simulink model "scouts"  (R2018a)
settings: Solver=VariableStepAuto  StartTime=0.0  StopTime=500  FixedStep=0.01  MaxStep=0.01  RelTol=1e-5
undefined symbols (not defined in the file or in its folder): sigbuilder_block
libraries: simulink x2
settings Model: Creator=daniel  LastModifiedBy=blond
settings SolverCC: ZeroCrossAlgorithm=Adaptive  AlgebraicLoopSolver=LineSearch
settings DebuggingCC: MaxConsecutiveZCsMsg=warning

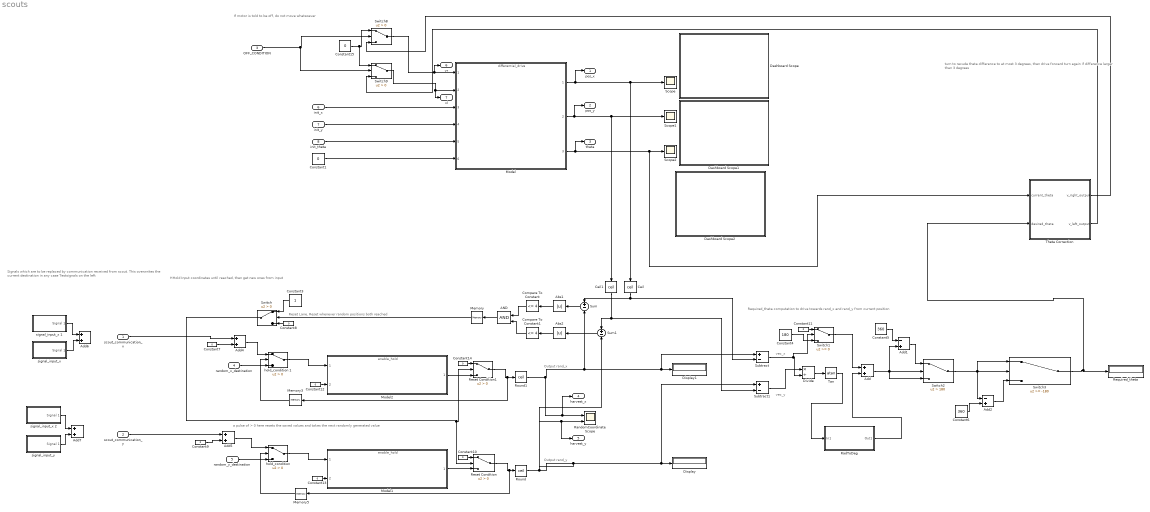
== system scouts ==
  note: If motor is told to be off, do not move whatsoever
  note: Signals which are to be replaced
      | by communication received
      | from scout. This overwrites the
      | current destination in any case
      |
      | Testsignals on the left
  note: turn to recude theta difference to at
      | most 3 degrees, then drive forward
      | turn again if difference larger than
      | 3 degrees
  note: Required_theta computation to drive towards rand_x and rand_y from current position
  note: vec_y
  note: Reset Lane, Reset whenever random positions both reached
  note: a pulse of > 0 here resets the saved values and takes the next randomly generated value
  note: Output rand_x
  note: HHold Input coordinates until reached, then get new ones from input
  note: Output rand_y
  note: vec_x
  "scout_communication_x " : Inport
  scout_communication_y : Inport  Port=2
  "OFF_CONDITION " : Inport  Port=3
  random_x_destination : Inport  Port=4
  random_y_destination : Inport  Port=5
  "init_x " : Inport  Port=6
  init_y : Inport  Port=7
  "init_theta " : Inport  Port=8
  AND : Logic  IconShape=distinctive  AllPortsSameDT=off  OutDataTypeStr=boolean
  Abs1 : Abs
  Abs2 : Abs
  Add{,4..7} (5 alike) : Sum
  Add1 : Sum  Inputs=-+
  Add2 : Sum  Inputs=-+
  Ceil : Rounding  Operator=ceil
  Ceil1 : Rounding  Operator=ceil
  Compare To Constant : simulink/Logic and Bit Operations/Compare To Constant  relop=<=  const=4  OutDataTypeStr=boolean
  Compare To Constant1 : simulink/Logic and Bit Operations/Compare To Constant  relop=<=  const=4  OutDataTypeStr=boolean
  Constant{1,7..15} (10 alike) : Constant  Value=0
  Constant3 : Constant
  Constant4 : Constant  Value=180
  Constant5 : Constant  Value=360
  Constant6 : Constant  Value=360
  Dashboard Scope : Subsystem  DialogController=hmiCreateDDGDialog  IsWebBlock=on  mask(MWDashboardBlock){webBlockId=28513450-4590-42fc-ab75-f58e69578865, webBlockType=sdiscope, ShowInitialText=on, HMISrcModelName=scouts}
      mask prompts: webBlockId "WebBlock Id"; webBlockType "WebBlock Type"; HMISrcModelName "Source Model"
      mask help: SimulinkHMI:dialogs:HMIScopeDialogDesc
      mask Help: helpview([docroot '/mapfiles/simulink.map'], 'hmi_scope')
      mask Display:
      | if strcmp(get_param(bdroot(gcb),'BlockDiagramType'), 'library')
      |     image([(matlabroot) '/toolbox/simulink/hmi/icons/DashboardScope.png']);
      | end
  Dashboard Scope1 : Subsystem  DialogController=hmiCreateDDGDialog  IsWebBlock=on  mask(MWDashboardBlock){webBlockId=3c51b7a5-38a5-4713-bbf7-871b8fd5eea3, webBlockType=sdiscope, ShowInitialText=on, HMISrcModelName=scouts}
      mask prompts: webBlockId "WebBlock Id"; webBlockType "WebBlock Type"; HMISrcModelName "Source Model"
      mask help: SimulinkHMI:dialogs:HMIScopeDialogDesc
      mask Help: helpview([docroot '/mapfiles/simulink.map'], 'hmi_scope')
      mask Display:
      | if strcmp(get_param(bdroot(gcb),'BlockDiagramType'), 'library')
      |     image([(matlabroot) '/toolbox/simulink/hmi/icons/DashboardScope.png']);
      | end
  Dashboard Scope2 : Subsystem  DialogController=hmiCreateDDGDialog  IsWebBlock=on  mask(MWDashboardBlock){webBlockId=0047718c-4f1b-48ee-af11-e80bd18439e0, webBlockType=sdiscope, ShowInitialText=on, HMISrcModelName=scouts}
      mask prompts: webBlockId "WebBlock Id"; webBlockType "WebBlock Type"; HMISrcModelName "Source Model"
      mask help: SimulinkHMI:dialogs:HMIScopeDialogDesc
      mask Help: helpview([docroot '/mapfiles/simulink.map'], 'hmi_scope')
      mask Display:
      | if strcmp(get_param(bdroot(gcb),'BlockDiagramType'), 'library')
      |     image([(matlabroot) '/toolbox/simulink/hmi/icons/DashboardScope.png']);
      | end
  Display : Display
  Display1 : Display
  Divide : Product  Inputs=*/
  Memory : Memory
  Memory3 : Memory  InheritSampleTime=on
  Memory5 : Memory  InheritSampleTime=on
  Model : ModelReference  ModelNameDialog=differential_drive.slx  SimulationMode=Normal  ModelReferenceVersion=1.286
  Model1 : ModelReference  ModelNameDialog=enable_hold.slx  SimulationMode=Normal  ModelReferenceVersion=1.281
  Model2 : ModelReference  ModelNameDialog=enable_hold.slx  SimulationMode=Normal  ModelReferenceVersion=1.281
  RadToDeg : Subsystem
  "RandomCoordinate Scope " : Scope  NumInputPorts=2
  Required_theta : Display
  Reset Condition : Switch  Criteria=u2 > Threshold
  Reset Condition1 : Switch  Criteria=u2 > Threshold
  Round : Rounding  Operator=ceil
  Round1 : Rounding  Operator=ceil
  Scope : Scope
  Scope1 : Scope
  Scope2 : Scope
  Subtract : Sum  Inputs=+-
  Subtract1 : Sum  Inputs=+-
  Sum : Sum  Inputs=+-
  Sum1 : Sum  Inputs=+-
  Switch : Switch  Criteria=u2 > Threshold
  Switch1 : Switch
  Switch2 : Switch  Criteria=u2 > Threshold  Threshold=180
  Switch3 : Switch  Threshold=-180
  Switch8 : Switch  Criteria=u2 > Threshold
  Switch9 : Switch  Criteria=u2 > Threshold
  Tan : Trigonometry  Operator=atan  OutputSignalType=real
  "Theta Correction " : Subsystem
  "hold_condition " : Switch  Criteria=u2 > Threshold
  hold_condition 1 : Switch  Criteria=u2 > Threshold
  "signal_input_x " : Subsystem  Tag=STV Subsys  LoadFcn=sigbuilder_block('load');  StartFcn=sigbuilder_block('start');  StopFcn=sigbuilder_block('stop');  ClipboardFcn=sigbuilder_block('clipboard');  mask(Sigbuilder block){tuvar=[0:10]}
      mask help: Simulink:masks:SigbuilderBlock_MD
      mask init:
      | if ~strcmp(get_param(bdroot(gcbh),'SimulationStatus'),'stopped') tuvar = sigbuilder_block('maskInit'); end
      settings: CopyFcn=sigbuilder_block('copy');  DeleteFcn=sigbuilder_block('delete');  ModelCloseFcn=sigbuilder_block('modelClose');  PreSaveFcn=sigbuilder_block('preSave');  PauseFcn=sigbuilder_block('pause');  ContinueFcn=sigbuilder_block('continue');  NameChangeFcn=sigbuilder_block('namechange');  OpenFcn=sigbuilder_block('open',[441 370 550 400 ]);  CloseFcn=sigbuilder_block('close');
      mask Display: plot(0, 0, 100, 100,[2, 2, 32, 32, 2], [68, 8, 8, 68, 68],[32, 2], [38, 38], [32, 19, 2],[53, 60, 44], [32, 17, 17, 2],[16, 16, 31, 31]);txt = getActiveGroup(gcbh);text(2, 100, txt,'verticalAlignment', 'top');
  signal_input_x 1 : Subsystem  Tag=STV Subsys  LoadFcn=sigbuilder_block('load');  StartFcn=sigbuilder_block('start');  StopFcn=sigbuilder_block('stop');  ClipboardFcn=sigbuilder_block('clipboard');  mask(Sigbuilder block){tuvar=[0:10]}
      mask help: Simulink:masks:SigbuilderBlock_MD
      mask init:
      | if ~strcmp(get_param(bdroot(gcbh),'SimulationStatus'),'stopped') tuvar = sigbuilder_block('maskInit'); end
      settings: CopyFcn=sigbuilder_block('copy');  DeleteFcn=sigbuilder_block('delete');  ModelCloseFcn=sigbuilder_block('modelClose');  PreSaveFcn=sigbuilder_block('preSave');  PauseFcn=sigbuilder_block('pause');  ContinueFcn=sigbuilder_block('continue');  NameChangeFcn=sigbuilder_block('namechange');  OpenFcn=sigbuilder_block('open',[441 370 550 400 ]);  CloseFcn=sigbuilder_block('close');
      mask Display: plot(0, 0, 100, 100,[2, 2, 32, 32, 2], [68, 8, 8, 68, 68],[32, 2], [38, 38], [32, 19, 2],[53, 60, 44], [32, 17, 17, 2],[16, 16, 31, 31]);txt = getActiveGroup(gcbh);text(2, 100, txt,'verticalAlignment', 'top');
  signal_input_x 2 : Subsystem  Tag=STV Subsys  LoadFcn=sigbuilder_block('load');  StartFcn=sigbuilder_block('start');  StopFcn=sigbuilder_block('stop');  ClipboardFcn=sigbuilder_block('clipboard');  mask(Sigbuilder block){tuvar=[0:10]}
      mask help: Simulink:masks:SigbuilderBlock_MD
      mask init:
      | if ~strcmp(get_param(bdroot(gcbh),'SimulationStatus'),'stopped') tuvar = sigbuilder_block('maskInit'); end
      settings: CopyFcn=sigbuilder_block('copy');  DeleteFcn=sigbuilder_block('delete');  ModelCloseFcn=sigbuilder_block('modelClose');  PreSaveFcn=sigbuilder_block('preSave');  PauseFcn=sigbuilder_block('pause');  ContinueFcn=sigbuilder_block('continue');  NameChangeFcn=sigbuilder_block('namechange');  OpenFcn=sigbuilder_block('open',[441 370 550 400 ]);  CloseFcn=sigbuilder_block('close');
      mask Display: plot(0, 0, 100, 100,[2, 2, 32, 32, 2], [68, 8, 8, 68, 68],[32, 2], [38, 38], [32, 19, 2],[53, 60, 44], [32, 17, 17, 2],[16, 16, 31, 31]);txt = getActiveGroup(gcbh);text(2, 100, txt,'verticalAlignment', 'top');
  "signal_input_y " : Subsystem  Tag=STV Subsys  LoadFcn=sigbuilder_block('load');  StartFcn=sigbuilder_block('start');  StopFcn=sigbuilder_block('stop');  ClipboardFcn=sigbuilder_block('clipboard');  mask(Sigbuilder block){tuvar=[0:10]}
      mask help: Simulink:masks:SigbuilderBlock_MD
      mask init:
      | if ~strcmp(get_param(bdroot(gcbh),'SimulationStatus'),'stopped') tuvar = sigbuilder_block('maskInit'); end
      settings: CopyFcn=sigbuilder_block('copy');  DeleteFcn=sigbuilder_block('delete');  ModelCloseFcn=sigbuilder_block('modelClose');  PreSaveFcn=sigbuilder_block('preSave');  PauseFcn=sigbuilder_block('pause');  ContinueFcn=sigbuilder_block('continue');  NameChangeFcn=sigbuilder_block('namechange');  OpenFcn=sigbuilder_block('open',[348 215 550 400 ]);  CloseFcn=sigbuilder_block('close');
      mask Display: plot(0, 0, 100, 100,[2, 2, 32, 32, 2], [68, 8, 8, 68, 68],[32, 2], [38, 38], [32, 19, 2],[53, 60, 44], [32, 17, 17, 2],[16, 16, 31, 31]);txt = getActiveGroup(gcbh);text(2, 100, txt,'verticalAlignment', 'top');
  pos_x : Outport
  pos_y : Outport  Port=2
  theta : Outport  Port=3
  harvest_x : Outport  Port=4
  harvest_y : Outport  Port=5
  vr : Outport  Port=6
  vl : Outport  Port=7
  wires:
  "init_theta "/1 -> Model/5
  init_y/1 -> Model/4
  "init_x "/1 -> Model/3
  Model/1 -> pos_x/1, Scope/1, Ceil/1
  Model/2 -> pos_y/1, Scope1/1, Ceil1/1
  Model/3 -> theta/1, "Theta Correction "/1(current_theta), Scope2/1
  Constant1/1 -> Model/6
  random_y_destination/1 -> "hold_condition "/3
  "hold_condition "/1 -> Model1/1
  Round/1 -> harvest_y/1, "RandomCoordinate Scope "/2, Sum1/2, Subtract1/1, Display/1
  Model1/1 -> Reset Condition/3
  Round1/1 -> harvest_x/1, "RandomCoordinate Scope "/1, Subtract/1, Display1/1, Sum/2
  Model2/1 -> Reset Condition1/3
  hold_condition 1/1 -> Model2/1
  random_x_destination/1 -> hold_condition 1/3
  Compare To Constant/1 -> AND/1
  Compare To Constant1/1 -> AND/2
  Ceil1/1 -> Sum1/1, Subtract1/2
  Ceil/1 -> Sum/1, Subtract/2
  AND/1 -> Memory/1
  Constant3/1 -> Switch/1
  Memory/1 -> Switch/2
  Switch/1 -> Reset Condition/2, Reset Condition1/2
  Subtract1/1 -> Divide/1
  Subtract/1 -> Switch1/2, Divide/2
  Divide/1 -> Tan/1
  Tan/1 -> RadToDeg/1(In1)
  Switch1/1 -> Add/1
  Constant4/1 -> Switch1/3
  Add/1 -> Switch2/3, Switch2/2, Add1/2
  Constant5/1 -> Add1/1
  Add1/1 -> Switch2/1
  Switch2/1 -> Switch3/1, Switch3/2, Add2/1
  Constant6/1 -> Add2/2
  Add2/1 -> Switch3/3
  Switch3/1 -> "Theta Correction "/2(desired_theta), Required_theta/1
  RadToDeg/1(Out1) -> Add/2
  "Theta Correction "/1(v_right_output) -> Switch8/3
  "Theta Correction "/2(v_left_output) -> Switch9/3
  Constant7/1 -> Add4/2
  Constant8/1 -> Switch/3
  Constant10/1 -> Reset Condition/1
  Constant11/1 -> Switch1/1
  Constant12/1 -> Model2/2
  Constant13/1 -> Model1/2
  Constant14/1 -> Reset Condition1/1
  Reset Condition1/1 -> Memory3/1, Round1/1
  Reset Condition/1 -> Memory5/1, Round/1
  Sum/1 -> Abs1/1
  Abs1/1 -> Compare To Constant/1
  Abs2/1 -> Compare To Constant1/1
  Sum1/1 -> Abs2/1
  Memory5/1 -> "hold_condition "/2
  Memory3/1 -> hold_condition 1/2
  Add4/1 -> hold_condition 1/1
  Constant9/1 -> Add5/2
  Add5/1 -> "hold_condition "/1
  "signal_input_y "/1(Signal 1) -> Add7/2
  "signal_input_x "/1(Signal 1) -> Add6/2
  signal_input_x 2/1(Signal 1) -> Add7/1
  signal_input_x 1/1(Signal 1) -> Add6/1
  "scout_communication_x "/1 -> Add4/1
  scout_communication_y/1 -> Add5/1
  "OFF_CONDITION "/1 -> Switch9/2, Switch8/2
  Constant15/1 -> Switch9/1, Switch8/1
  Switch8/1 -> Model/1, vr/1
  Switch9/1 -> Model/2, vl/1

== system scouts/Dashboard Scope ==

== system scouts/Dashboard Scope1 ==

== system scouts/Dashboard Scope2 ==

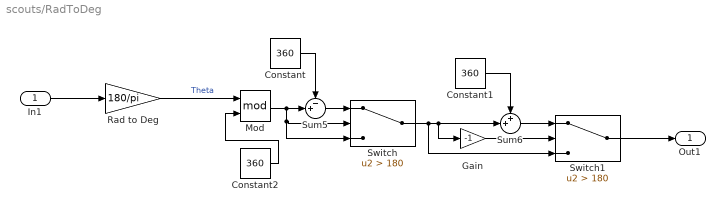
== system scouts/RadToDeg ==
  In1 : Inport
  Constant : Constant  Value=360
  Constant1 : Constant  Value=360
  Constant2 : Constant  Value=360
  Gain : Gain  Gain=-1
  Mod : Math  Operator=mod  SaturateOnIntegerOverflow=on
  Rad to Deg : Gain  Gain=180/pi
  Sum5 : Sum  Inputs=-+|
  Sum6 : Sum  Inputs=++|
  Switch : Switch  Criteria=u2 > Threshold  Threshold=180
  Switch1 : Switch  Criteria=u2 > Threshold  Threshold=180
  Out1 : Outport
  wires:
  Constant/1 -> Sum5/1
  Constant1/1 -> Sum6/1
  Rad to Deg/1 -> Mod/1  "Theta"
  Gain/1 -> Switch1/2
  Switch/1 -> Sum6/2, Gain/1, Switch1/3
  Sum5/1 -> Switch/1
  Mod/1 -> Sum5/2, Switch/2, Switch/3
  Sum6/1 -> Switch1/1
  Constant2/1 -> Mod/2
  In1/1 -> Rad to Deg/1
  Switch1/1 -> Out1/1

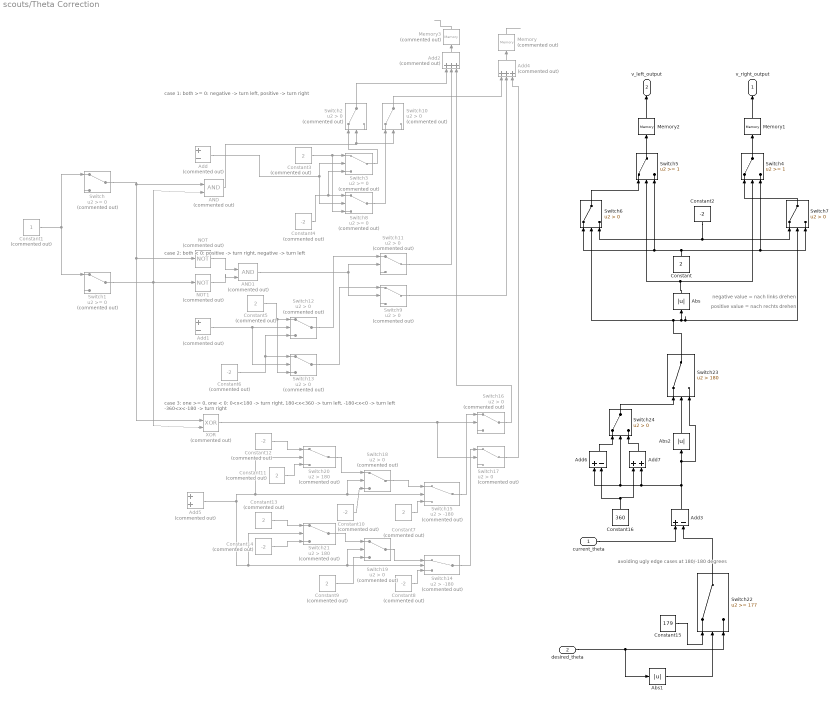
== system scouts/Theta Correction  ==
  note: avoiding ugly edge cases at
      | 180/-180 degrees
  note: case 3: one >= 0, one < 0:   0<x<180 -> turn right,  180<x<360 -> turn left,
      |                                               -180<x<0 -> turn left   -360<x<-180 -> turn right
  note: case 2: both < 0: positive -> turn right, negative -> turn left
  note: case 1: both >= 0: negative -> turn left, positive -> turn right
  note: positive value = nach rechts drehen
  note: negative value = nach links drehen
  current_theta : Inport
  desired_theta : Inport  Port=2
  AND : Logic  Commented=on  IconShape=distinctive  AllPortsSameDT=off  OutDataTypeStr=boolean
  AND1 : Logic  Commented=on  IconShape=distinctive  AllPortsSameDT=off  OutDataTypeStr=boolean
  Abs : Abs
  Abs1 : Abs
  Abs2 : Abs
  Add : Sum  Commented=on  Inputs=+-
  Add1 : Sum  Commented=on  Inputs=+-
  Add2 : Sum  Commented=on  Inputs=+++
  Add3 : Sum  Inputs=+-
  Add4 : Sum  Commented=on  Inputs=+++
  Add5 : Sum  Commented=on
  Add6 : Sum  Inputs=+-
  Add7 : Sum
  Constant : Constant  Value=2
  Constant1 : Constant  Commented=on
  Constant{4,6,8,10,12,14} (6 alike) : Constant  Commented=on  Value=-2
  Constant{3,5,7,9,11,13} (6 alike) : Constant  Commented=on  Value=2
  Constant15 : Constant  Value=179
  Constant16 : Constant  Value=360
  Constant2 : Constant  Value=-2
  Memory : Memory  Commented=on
  Memory1 : Memory
  Memory2 : Memory
  Memory3 : Memory  Commented=on
  NOT : Logic  Commented=on  Operator=NOT  IconShape=distinctive  AllPortsSameDT=off  OutDataTypeStr=boolean
  NOT1 : Logic  Commented=on  Operator=NOT  IconShape=distinctive  AllPortsSameDT=off  OutDataTypeStr=boolean
  Switch{,1,3,8} (4 alike) : Switch  Commented=on
  Switch{2,9..13,16..19} (10 alike) : Switch  Commented=on  Criteria=u2 > Threshold
  Switch14 : Switch  Commented=on  Criteria=u2 > Threshold  Threshold=-180
  Switch15 : Switch  Commented=on  Criteria=u2 > Threshold  Threshold=-180
  Switch20 : Switch  Commented=on  Criteria=u2 > Threshold  Threshold=180
  Switch21 : Switch  Commented=on  Criteria=u2 > Threshold  Threshold=180
  Switch22 : Switch  Threshold=177
  Switch23 : Switch  Criteria=u2 > Threshold  Threshold=180
  Switch24 : Switch  Criteria=u2 > Threshold
  Switch4 : Switch  Threshold=1
  Switch5 : Switch  Threshold=1
  Switch6 : Switch  Criteria=u2 > Threshold
  Switch7 : Switch  Criteria=u2 > Threshold
  XOR : Logic  Commented=on  Operator=XOR  IconShape=distinctive  AllPortsSameDT=off  OutDataTypeStr=boolean
  v_right_output : Outport
  v_left_output : Outport  Port=2
  wires:
  desired_theta/1 -> Switch22/3, Abs1/1
  current_theta/1 -> Add3/1
  Memory2/1 -> v_left_output/1
  Switch6/1 -> Switch5/1
  Switch4/1 -> Memory1/1
  Switch7/1 -> Switch4/1
  Switch5/1 -> Memory2/1
  Abs/1 -> Switch4/2, Switch5/2
  Constant2/1 -> Switch7/1, Switch6/3
  Switch23/1 -> Abs/1, Switch7/2, Switch6/2
  Constant/1 -> Switch7/3, Switch4/3, Switch6/1, Switch5/3
  Memory1/1 -> v_right_output/1
  ? -> Add5/1, Add1/1, Add/1, Switch/2
  ? -> Add1/2, Add5/2, Switch1/2, Add/2
  Constant1/1 -> Switch/1, Switch1/1
  Switch/1 -> XOR/1, NOT/1, AND/1
  Switch1/1 -> XOR/2, NOT1/1, AND/2
  Add/1 -> Switch8/2, Switch3/2
  Constant3/1 -> Switch8/3, Switch3/1
  Constant4/1 -> Switch3/3, Switch8/1
  NOT/1 -> AND1/1
  NOT1/1 -> AND1/2
  AND/1 -> Switch10/2, Switch2/2
  Switch3/1 -> Switch2/1
  Switch2/1 -> Add2/1
  Switch8/1 -> Switch10/1
  Switch10/1 -> Add4/1
  AND1/1 -> Switch9/2, Switch11/2
  Add2/1 -> Memory3/1
  Add4/1 -> Memory/1
  Switch11/1 -> Add2/2
  Switch9/1 -> Add4/2
  Add1/1 -> Switch13/2, Switch12/2
  Constant5/1 -> Switch13/3, Switch12/1
  Constant6/1 -> Switch13/1, Switch12/3
  Switch12/1 -> Switch11/1
  Switch13/1 -> Switch9/1
  Add5/1 -> Switch19/2, Switch14/2, Switch21/2, Switch20/2, Switch18/2, Switch15/2
  XOR/1 -> Switch17/2, Switch16/2
  Switch15/1 -> Switch16/1
  Switch14/1 -> Switch17/1
  Switch16/1 -> Add2/3
  Switch17/1 -> Add4/3
  Constant7/1 -> Switch15/3
  Constant8/1 -> Switch14/3
  Switch18/1 -> Switch15/1
  Switch19/1 -> Switch14/1
  Constant9/1 -> Switch19/3
  Constant10/1 -> Switch18/3
  Switch21/1 -> Switch19/1
  Switch20/1 -> Switch18/1
  Constant11/1 -> Switch20/3
  Constant12/1 -> Switch20/1
  Constant13/1 -> Switch21/1
  Constant14/1 -> Switch21/3
  Memory/1 -> ?
  Memory3/1 -> ?
  Abs1/1 -> Switch22/2
  Switch22/1 -> Add3/2
  Constant15/1 -> Switch22/1
  Add3/1 -> Add7/2, Add6/1, Switch24/2, Switch23/3, Abs2/1
  Abs2/1 -> Switch23/2
  Add6/1 -> Switch24/1
  Constant16/1 -> Add6/2, Add7/1
  Add7/1 -> Switch24/3
  Switch24/1 -> Switch23/1

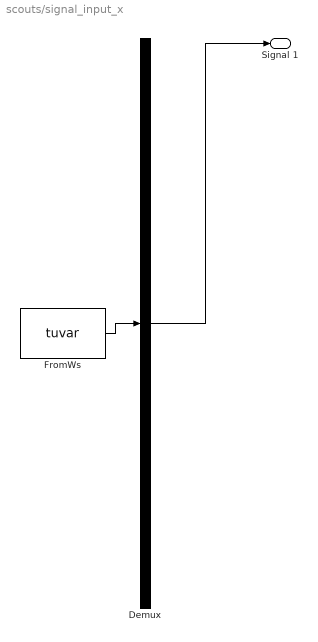
== system scouts/signal_input_x  ==
  Demux : Demux  Tag=STV Demux  Outputs=1
  FromWs : FromWorkspace  Tag=STV FromWs  VariableName=tuvar  SampleTime=0
      SigBuilderData=|
      | common.afterFinalStr = 'Extrapolate'
      | common.sampleTime = 0
      | dataSet.timeRange = [0 100]
      | dataSet.name = 'Group 1'
      | sbobj.Groups.Name = 'Group 1'
      | sbobj.Groups.Signals.Name = 'Signal 1'
      | sbobj.Groups.Signals.XData = [0 49.9 49.9 50 50 100]
      | sbobj.Groups.Signals.YData = [0 0 199 199 0 0]
      | sbobj.Groups.TimeRange = [0 100]
  Signal 1 : Outport  Tag=STV Outport
  wires:
  Demux/1 -> Signal 1/1
  FromWs/1 -> Demux/1

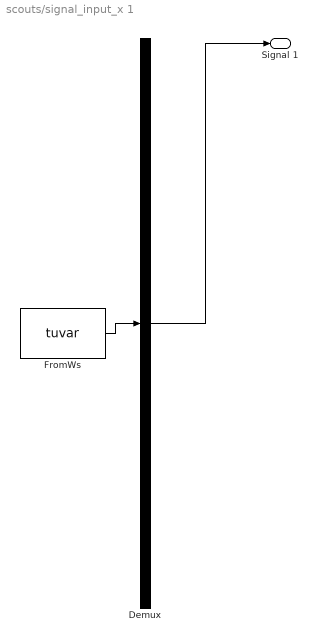
== system scouts/signal_input_x 1 ==
  Demux : Demux  Tag=STV Demux  Outputs=1
  FromWs : FromWorkspace  Tag=STV FromWs  VariableName=tuvar  SampleTime=0
      SigBuilderData=|
      | common.afterFinalStr = 'Extrapolate'
      | common.sampleTime = 0
      | dataSet.timeRange = [0 200]
      | dataSet.name = 'Group 1'
      | sbobj.Groups.Name = 'Group 1'
      | sbobj.Groups.Signals.Name = 'Signal 1'
      | sbobj.Groups.Signals.XData = [0 99.9 99.9 100 100 200]
      | sbobj.Groups.Signals.YData = [0 0 1 1 0 0]
      | sbobj.Groups.TimeRange = [0 200]
  Signal 1 : Outport  Tag=STV Outport
  wires:
  Demux/1 -> Signal 1/1
  FromWs/1 -> Demux/1

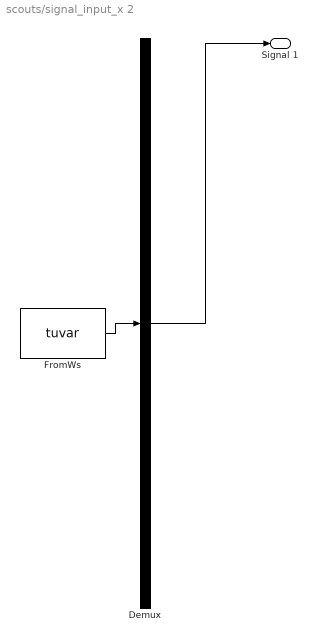
== system scouts/signal_input_x 2 ==
  Demux : Demux  Tag=STV Demux  Outputs=1
  FromWs : FromWorkspace  Tag=STV FromWs  VariableName=tuvar  SampleTime=0
      SigBuilderData=|
      | common.afterFinalStr = 'Extrapolate'
      | common.sampleTime = 0
      | dataSet.timeRange = [0 200]
      | dataSet.name = 'Group 1'
      | sbobj.Groups.Name = 'Group 1'
      | sbobj.Groups.Signals.Name = 'Signal 1'
      | sbobj.Groups.Signals.XData = [0 99.9 99.9 100 100 200]
      | sbobj.Groups.Signals.YData = [0 0 1 1 0 0]
      | sbobj.Groups.TimeRange = [0 200]
  Signal 1 : Outport  Tag=STV Outport
  wires:
  Demux/1 -> Signal 1/1
  FromWs/1 -> Demux/1

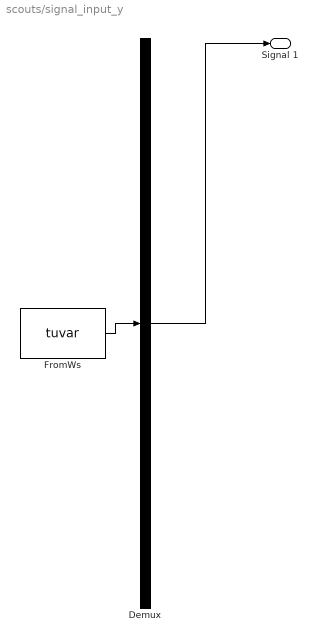
== system scouts/signal_input_y  ==
  Demux : Demux  Tag=STV Demux  Outputs=1
  FromWs : FromWorkspace  Tag=STV FromWs  VariableName=tuvar  SampleTime=0
      SigBuilderData=|
      | common.afterFinalStr = 'Extrapolate'
      | common.sampleTime = 0
      | dataSet.timeRange = [0 100]
      | dataSet.name = 'Group 1'
      | sbobj.Groups.Name = 'Group 1'
      | sbobj.Groups.Signals.Name = 'Signal 1'
      | sbobj.Groups.Signals.XData = [0 49.9 49.9 50 50 100]
      | sbobj.Groups.Signals.YData = [0 0 99 99 0 0]
      | sbobj.Groups.TimeRange = [0 100]
  Signal 1 : Outport  Tag=STV Outport
  wires:
  Demux/1 -> Signal 1/1
  FromWs/1 -> Demux/1
